simulink model "HANcoder_E407_KinematicAngleControl"  (R2022a)
settings: Solver=FixedStepDiscrete  StartTime=0.0  StopTime=1  FixedStep=0.01  RelTol=1e-3
PreLoadFcn:
  | librarySetup
  | eval([bdroot,'_startup']) %Calling [modelName]_startup.m
values from neighbouring files (symbols this model uses):
  L0b = 1    [HANcoder_E407_KinematicAngleControl_startup.m]    (also in HANcoder_E407_TTA_CombineModel_Membership_2022a_startup.m; HANcoder_E407_TTA_CombineModel_Membership_startup.m; HANcoder_E407_TTA_CombineModel_V2_startup.m; HANcoder_E407_TTA_CombineModel_startup.m)
  L0F = 3    [HANcoder_E407_KinematicAngleControl_startup.m]    (also in HANcoder_E407_TTA_CombineModel_Membership_2022a_startup.m; HANcoder_E407_TTA_CombineModel_Membership_startup.m; HANcoder_E407_TTA_CombineModel_V2_startup.m; HANcoder_E407_TTA_CombineModel_startup.m)
  L1F = 4    [HANcoder_E407_KinematicAngleControl_startup.m]    (also in HANcoder_E407_TTA_CombineModel_Membership_2022a_startup.m; HANcoder_E407_TTA_CombineModel_Membership_startup.m; HANcoder_E407_TTA_CombineModel_V2_startup.m; HANcoder_E407_TTA_CombineModel_startup.m)
  V2 = 1.3889    [HANcoder_E407_KinematicAngleControl_startup.m]    (also in HANcoder_E407_TTA_CombineModel_Membership_2022a_startup.m = 0.5; HANcoder_E407_TTA_CombineModel_Membership_startup.m = 0.5; HANcoder_E407_TTA_CombineModel_V2_startup.m = 0.5; HANcoder_E407_TTA_CombineModel_startup.m)
undefined symbols (not defined in the file or in its folder): A1, A2, A3, A4, A5, CON2, CON3, D4, D5
libraries: HANcoder_STM32_Target x14, slpidlib x1, simulink x1
settings Model: Creator=Jason van Kolfschoten  LastModifiedBy=lenovo
settings SolverCC: AlgebraicLoopSolver=TrustRegion  PositivePriorityOrder=on
settings DataIOCC: LimitDataPoints=on  SaveFormat=Array  SignalLoggingSaveFormat=ModelDataLogs  SaveOutput=off  SignalLogging=off  DSMLogging=off  SaveTime=off  ReturnWorkspaceOutputs=off
settings OptimizationCC: BlockReduction=off  DefaultParameterBehavior=Inlined  DefaultUnderspecifiedDataType=single  InlineInvariantSignals=on  ExpressionDepthLimit=2147483647  StateBitsets=on  DataBitsets=on  ZeroExternalMemoryAtStartup=off  ZeroInternalMemoryAtStartup=off  InitFltsAndDblsToZero=on  NoFixptDivByZeroProtection=on  EfficientFloat2IntCast=on  LifeSpan=inf  EfficientTunableParamExpr=on
settings DebuggingCC: SaveWithDisabledLinksMsg=none  SaveWithParameterizedLinksMsg=none  CheckSSInitialOutputMsg=off  UnderspecifiedInitializationDetection=Classic  MergeDetectMultiDrivingBlocksExec=none  SignalResolutionControl=TryResolveAll  SolverPrmCheckMsg=warning  InheritedTsInSrcMsg=none  MultiTaskDSMMsg=warning  MultiTaskCondExecSysMsg=none  ParameterPrecisionLossMsg=none  FcnCallInpInsideContextMsg=warning  UnconnectedInputMsg=warning  UnconnectedOutputMsg=warning  UnconnectedLineMsg=warning  StateNameClashWarn=warning  SFUnexpectedBacktrackingDiag=warning  SFNoUnconditionalDefaultTransitionDiag=warning  SFExecutionAtInitializationDiag=none  SFMachineParentedDataDiag=warning  ArithmeticOperatorsInVariantConditions=warning
settings HardwareCC: ProdBitPerPointer=32  ProdBitPerSizeT=32  ProdBitPerPtrDiffT=32  ProdLargestAtomicInteger=Long  ProdLargestAtomicFloat=Double  ProdWordSize=32  ProdHWDeviceType=ARM Compatible->ARM Cortex  TargetEndianess=LittleEndian  TargetHWDeviceType=Infineon->TriCore
settings ModelReferenceCC: PropagateSignalLabelsOutOfModel=off
settings SFSimCC: SimUseLocalCustomCode=off  MATLABDynamicMemAlloc=off  CustomCodeUndefinedFunction=UseInterfaceOnly
settings RTWCC: Description=Real-Time Workshop Embedded Coder (no auto configuration)  SystemTargetFile=ert.tlc  MakeCommand=make_rtw SHELL= HANcoder_PORTABLE=1 HANcoder_BOOTLOADER=1  TemplateMakefile=STM32_E407_gcc.tmf  RTWUseLocalCustomCode=off
settings CodeAppCC: ForceParamTrailComments=on  IgnoreCustomStorageClasses=off  SimulinkDataObjDesc=on  CustomSymbolStrGlobalVar=rt$N$M  CustomSymbolStrType=$N$M  CustomSymbolStrFcn=$N$M$F  CustomSymbolStrMacro=$N$M  InsertBlockDesc=on  StateflowObjectComments=on  InternalIdentifier=Classic
settings ERTTargetCC: TargetFcnLib=ansi_tfl_tmw.mat  MultiwordLength=2048  IncludeMdlTerminateFcn=off  SuppressErrorStatus=on  SupportNonFinite=off  GenerateASAP2=on  InlinedParameterPlacement=NonHierarchical  ERTCustomFileTemplate=example_file_process.tlc  ConvertIfToSwitch=off  SuppressUnreachableDefaultCases=off
settings ConfigComp: CovMetricSettings=dw  CovSaveCumulativeToWorkspaceVar=on  CovSaveSingleToWorkspaceVar=on  CovExternalEMLEnable=off  CovSFcnEnable=off  DVMaxProcessTime=600  DVAutomaticStubbing=off  DVModelCoverageObjectives=MCDC  DVMaxTestCaseSteps=500  DVTestSuiteOptimization=CombinedObjectives  DVDetectActiveLogic=on  DVSaveHarnessModel=on  DVHarnessSource=Signal Editor

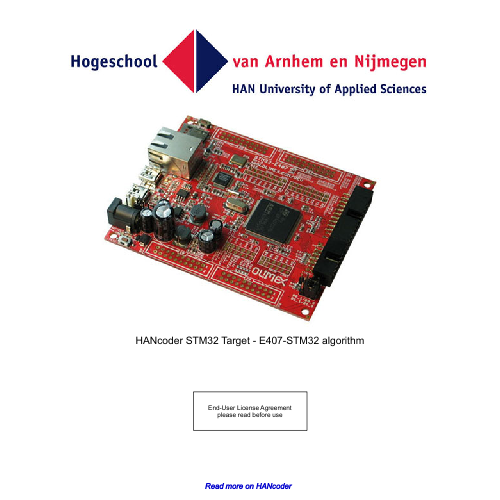
[thumbnail: Simulink's stored preview of the top-level diagram]
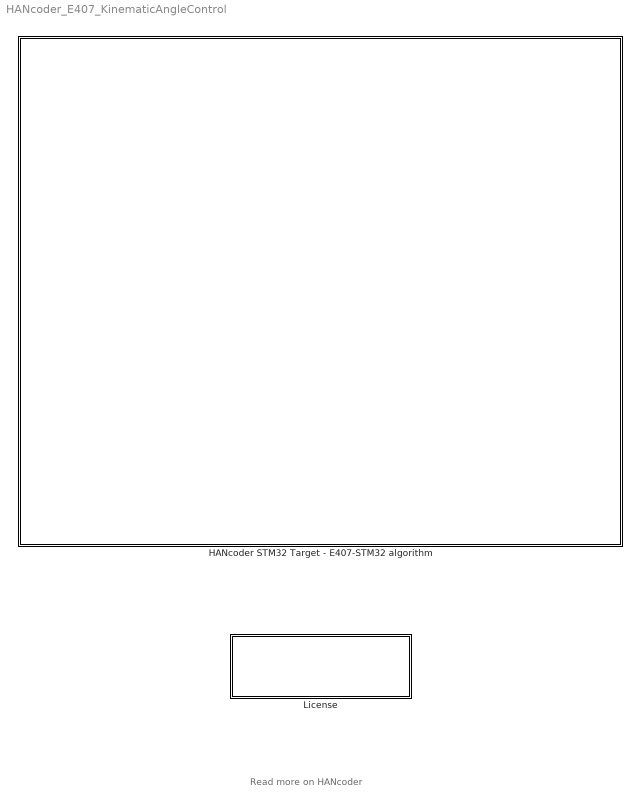
== system HANcoder_E407_KinematicAngleControl ==
  note: Read more on HANcoder
  HANcoder STM32 Target - E407-STM32 algorithm : Subsystem  mask(TopLevelSubsystem){}
      settings: CopyFcn=HANcoderChecks('Copy');  NameChangeFcn=HANcoderChecks('NameChangeE407');  MoveFcn=HANcoderChecks('MoveE407');
      mask Display: image(imread('STM32_E407_HAN.jpg'))
  License : Subsystem  mask(License){}
      settings: NameChangeFcn=HANcoderChecks('NameChangeLicenseBlock');  OpenFcn=winopen('License.pdf')  MoveFcn=HANcoderChecks('MoveLicenseBlock');
      mask Display: disp(['End-User License Agreement\n','please read before use']);

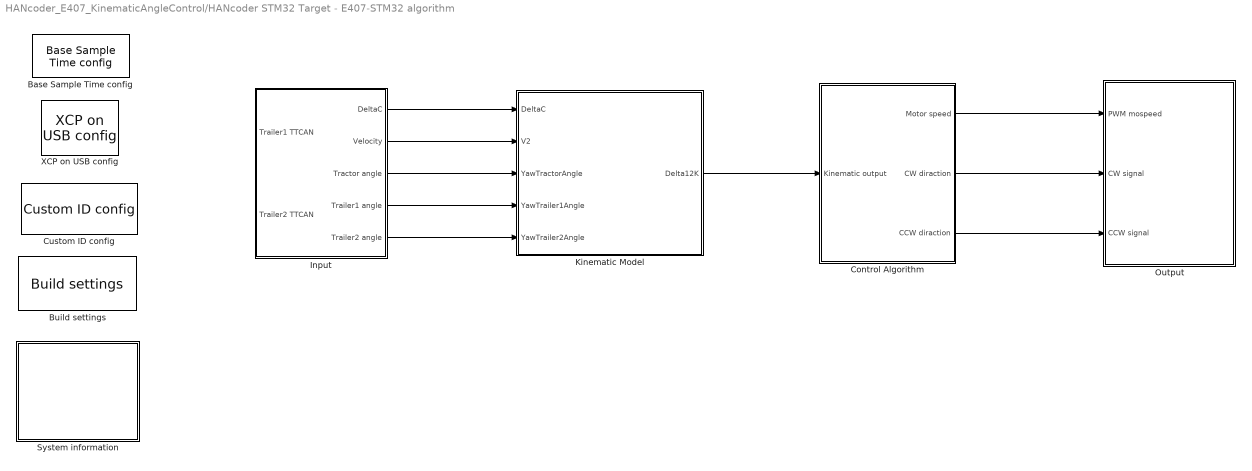
== system HANcoder_E407_KinematicAngleControl/HANcoder STM32 Target - E407-STM32 algorithm ==
  Base Sample Time config : HANcoder_STM32_Target/STM32-E407/System Config/Base Sample Time config  Tag=HANcoder_TARGET_STM32_E407  Description=HANcoder Target STM32-E407 blockset version 1.0  baseSampleTime=10  extraStack=100
      settings: SourceProductName=HANcoder STM32 Target
  Build settings : HANcoder_STM32_Target/STM32-E407/System Config/Build settings  Tag=HANcoder_TARGET_STM32_E407  AutoASAP2add=on  AutoFlash=USB
      settings: SourceProductName=HANcoder STM32 Target
  Control Algorithm : Subsystem
  Custom ID config : HANcoder_STM32_Target/STM32-E407/System Config/Custom ID config  Tag=HANcoder_TARGET_STM32_E407  softID=softwareID  softNUM=1
      settings: SourceProductName=HANcoder STM32 Target
  Input : Subsystem
  Kinematic Model : Subsystem
  "Output " : Subsystem
  System information : Subsystem
  XCP on USB config : HANcoder_STM32_Target/STM32-E407/System Config/XCP on USB config  Tag=HANcoder_TARGET_STM32_E407
      settings: SourceProductName=HANcoder STM32 Target
  wires:
  Input/1(DeltaC) -> Kinematic Model/1(DeltaC)
  Input/2(Velocity) -> Kinematic Model/2(V2)
  Input/3(Tractor angle) -> Kinematic Model/3(YawTractorAngle)
  Input/4(Trailer1 angle) -> Kinematic Model/4(YawTrailer1Angle)
  Input/5(Trailer2 angle) -> Kinematic Model/5(YawTrailer2Angle)
  Kinematic Model/1(Delta12K) -> Control Algorithm/1(Kinematic output)
  Control Algorithm/3(CCW diraction) -> "Output "/3(CCW signal)
  Control Algorithm/2(CW diraction) -> "Output "/2(CW signal)
  Control Algorithm/1(Motor speed) -> "Output "/1(PWM mospeed)

== system HANcoder_E407_KinematicAngleControl/License ==

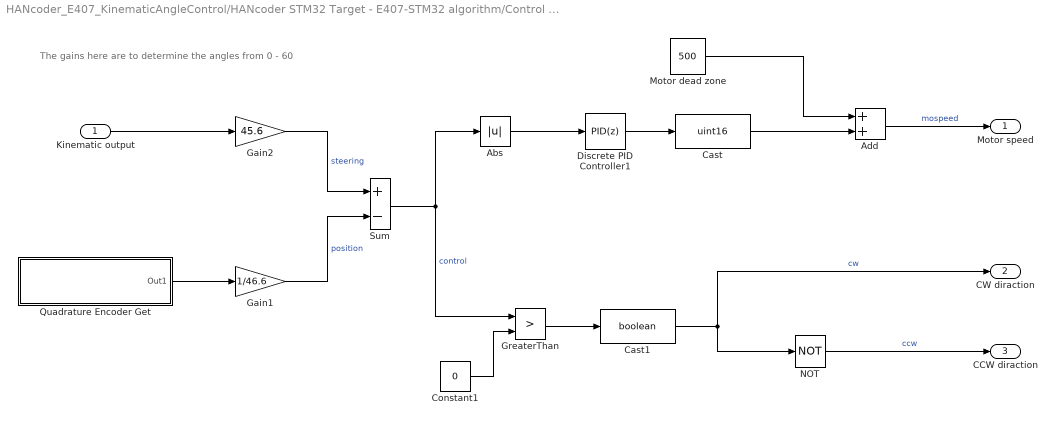
== system HANcoder_E407_KinematicAngleControl/HANcoder STM32 Target - E407-STM32 algorithm/Control Algorithm ==
  note: The gains here are to determine the angles from 0 - 60
  Kinematic output : Inport
  Abs : Abs  OutDataTypeStr=double  SaturateOnIntegerOverflow=off
  Add : Sum  AccumDataTypeStr=uint16
  Cast : DataTypeConversion  OutDataTypeStr=uint16  SaturateOnIntegerOverflow=off  RndMeth=Floor
  Cast1 : DataTypeConversion  OutDataTypeStr=boolean  SaturateOnIntegerOverflow=off  RndMeth=Floor
  Constant1 : Constant  Value=0
  Discrete PID Controller1 : slpidlib/PID Controller  Controller=PID  Form=Parallel  TimeDomain=Discrete-time  UseExternalTs=off  SampleTime=-1  IntegratorMethod=Forward Euler  FilterMethod=Forward Euler  ControllerParametersSource=internal  P=3  I=0.5  UseKiTs=off  D=0.5  N=100  UseFilter=on  TunerSelectOption=Transfer Function Based (PID Tuner App)  InitialConditionSource=internal  InitialConditionForIntegrator=0  InitialConditionForFilter=0  DifferentiatorICPrevScaledInput=0  ExternalReset=none  TrackingMode=off  Kt=1  LimitOutput=off  SatLimitsSource=internal  UpperSaturationLimit=inf  LowerSaturationLimit=-inf  LinearizeAsGain=off  AntiWindupMode=none  Kb=1  POutMin=[]  POutMax=[]  IOutMin=[]  IOutMax=[]  DOutMin=[]  DOutMax=[]  NOutMin=[]  NOutMax=[]  SumOutMin=[]  SumOutMax=[]  SaturationOutMin=[]  SaturationOutMax=[]  PParamMin=[]  PParamMax=[]  IParamMin=[]  IParamMax=[]  DParamMin=[]  DParamMax=[]  NParamMin=[]  NParamMax=[]  KbParamMin=[]  KbParamMax=[]  KtParamMin=[]  KtParamMax=[]  KbOutMin=[]  KbOutMax=[]  KtOutMin=[]  KtOutMax=[]  IntegratorOutMin=[]  IntegratorOutMax=[]  FilterOutMin=[]  FilterOutMax=[]  SumI1OutMin=[]  SumI1OutMax=[]  SumI2OutMin=[]  SumI2OutMax=[]  SumI3OutMin=[]  SumI3OutMax=[]  SumI4OutMin=[]  SumI4OutMax=[]  SumDOutMin=[]  SumDOutMax=[]  DifferentiatorOutMin=[]  DifferentiatorOutMax=[]  FilterDiffOutCoefMin=[]  FilterDiffOutCoefMax=[]  ReciprocalOutMin=[]  ReciprocalOutMax=[]  SumDenOutMin=[]  SumDenOutMax=[]  SumNumOutMin=[]  SumNumOutMax=[]  DivideOutMin=[]  DivideOutMax=[]  UdiffTsProdOutMin=[]  UdiffTsProdOutMax=[]  NTsProdOutMin=[]  NTsProdOutMax=[]  UintegralTsProdOutMin=[]  UintegralTsProdOutMax=[]  UngainTsProdOutMin=[]  UngainTsProdOutMax=[]  IntegratorContinuousStateAttributes=''  IntegratorStateMustResolveToSignalObject=off  IntegratorRTWStateStorageClass=Auto  FilterContinuousStateAttributes=''  FilterStateMustResolveToSignalObject=off  FilterRTWStateStorageClass=Auto  ParallelPVariant=InternalParameters  IdealPVariant=Disabled  IVariant=InternalParameters  DVariant=InternalParameters  IntegratorVariant=Discrete  SatVariant=Disabled  AWVariant=Passthrough  PCopyVariant=Disabled  TRVariant=Disabled  FdbkBlocksVariant=Forward  IdealPFdbkVariant=Disabled  SatFdbkVariant=Disabled  DerivativeFilterVariant=ForwardEulerFilter  NVariant=InternalParameters  NCopyVariant=Disabled  FilterICVariant=InternalICsFilter  IntegratorICVariant=InternalICs  ExternalResetVariant=Disabled  TRSumVariant=Passthrough  SumFdbkVariant=Disabled  SumVariant=Sum_PID  TsampFilterVariant=InternalTs  TsampNgainVariant=Passthrough  TsampIntegralVariant=Passthrough  ExternalSaturationOutDataTypeStr=Inherit: Same as second input  aMode=0
  Gain1 : Gain  Gain=1/46.6  OutDataTypeStr=double
  Gain2 : Gain  Gain=45.6
  GreaterThan : RelationalOperator  Operator=>  OutDataTypeStr=boolean  RndMeth=Simplest  InputSameDT=off
  Motor dead zone : Constant  Value=500  OutDataTypeStr=uint16
  NOT : Logic  Operator=NOT  IconShape=distinctive  AllPortsSameDT=off  OutDataTypeStr=boolean
  Quadrature Encoder Get : Subsystem  Tag=HANcoder_TARGET_STM32_E407  AncestorBlock=HANcoder_STM32_Target/STM32-E407/Timer Inputs/Quadrature Encoder Get  mask(Quadrature Encoder Inputs){moduleID=TIM3: CON4 - D12 & D11 (5V Tolerant), config=Floating, counterReset=off, tsamp=-1}
      mask prompts: moduleID "Quad encoder module"; config "Configuration"; counterReset "Show counter reset input"; tsamp "Sample time"
      mask help:
      | Function
      | ========
      | Reads the counter of the quadrature encoder module.
      |
      | Parameters
      | ==========
      | Quadrature encoder module:
      |   Selects the quadrature encoder module. The channel A and B signals of the
      |   encoder should be connected to the 2 input pins that belong to the module.
      |
      | Configuration:
      |   Determines if the input is floating or is connected to an internal
      |   pull-up or pull-down resistor.
      |
      | Show counter reset input:
      |   Configures if the input port for the counter reset should be shown.
      |
      |
      | Outport
      | ==========
      | 32-bit signed counter. The counter starts at zero and counts up or down
      | depending on the direction of the motor.
      mask init:
      | moduleIDInfoStr = sfcn_quad_encoder_get_mcb(2,moduleID, counterReset, config);
      settings: CopyFcn=sfcn_quad_encoder_get_chk();  MoveFcn=drawLogos
      mask Help: web('sfcn_quad_encoder_get.html');
      mask TypeOptions moduleID: TIM1: CON PE - 12 & 14 (5V Tolerant) | TIM3: CON4 - D12 & D11 (5V Tolerant) | TIM4: CON PD - 15 & 16 (5V Tolerant) | TIM8: UEXT - 3 & 4 (5V Tolerant)
      mask Callback moduleID: sfcn_quad_encoder_get_chk();
      mask TypeOptions config: Floating | Pullup | Pulldown
      mask Display: fprintf('Quad Encoder Get\n%s', moduleIDInfoStr);patch([135 141 141],[8 14 2],[1 0 0]);patch([143 143 149],[14 2 8],[0 0 0.35]);
  Sum : Sum  Inputs=+-
  Motor speed : Outport
  CW diraction : Outport  Port=2
  CCW diraction : Outport  Port=3
  wires:
  Motor dead zone/1 -> Add/1
  Sum/1 -> GreaterThan/1, Abs/1  "control"
  NOT/1 -> CCW diraction/1  "ccw"
  Abs/1 -> Discrete PID Controller1/1
  Cast/1 -> Add/2
  GreaterThan/1 -> Cast1/1
  Cast1/1 -> CW diraction/1, NOT/1  "cw"
  Add/1 -> Motor speed/1  "mospeed"
  Constant1/1 -> GreaterThan/2
  Gain1/1 -> Sum/2  "position"
  Discrete PID Controller1/1 -> Cast/1
  Quadrature Encoder Get/1(Out1) -> Gain1/1
  Gain2/1 -> Sum/1  "steering"
  Kinematic output/1 -> Gain2/1

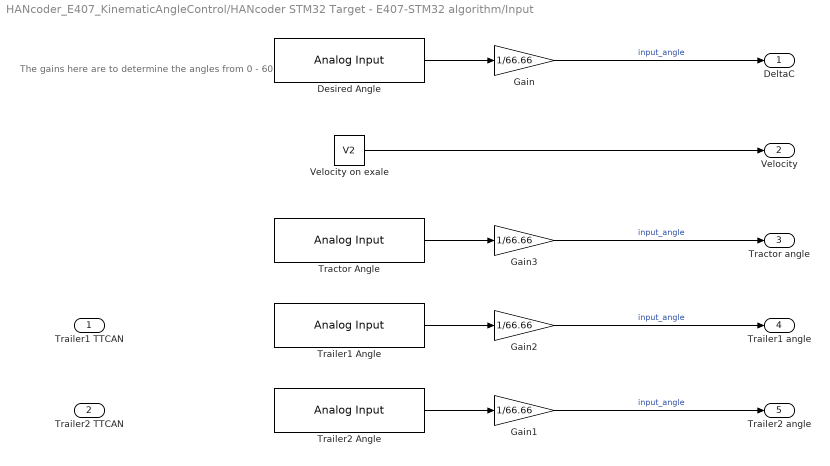
== system HANcoder_E407_KinematicAngleControl/HANcoder STM32 Target - E407-STM32 algorithm/Input ==
  note: The gains here are to determine the angles from 0 - 60
  Trailer1 TTCAN : Inport
  Trailer2 TTCAN : Inport  Port=2
  Desired Angle : HANcoder_STM32_Target/STM32-E407/Analog Inputs/Analog Input  Tag=HANcoder_TARGET_STM32_E407  pinID=CON2 - A1  tsamp=-1  filtered=off
      settings: SourceProductName=HANcoder STM32 Target
  Gain{,1..3} (4 alike) : Gain  Gain=1/66.66  OutDataTypeStr=double
  Tractor Angle : HANcoder_STM32_Target/STM32-E407/Analog Inputs/Analog Input  Tag=HANcoder_TARGET_STM32_E407  pinID=CON2 - A5  tsamp=-1  filtered=off
      settings: SourceProductName=HANcoder STM32 Target
  Trailer1 Angle : HANcoder_STM32_Target/STM32-E407/Analog Inputs/Analog Input  Tag=HANcoder_TARGET_STM32_E407  pinID=CON2 - A2  tsamp=-1  filtered=off
      settings: SourceProductName=HANcoder STM32 Target
  Trailer2 Angle : HANcoder_STM32_Target/STM32-E407/Analog Inputs/Analog Input  Tag=HANcoder_TARGET_STM32_E407  pinID=CON2 - A3  tsamp=-1  filtered=off
      settings: SourceProductName=HANcoder STM32 Target
  Velocity on exale : Constant  Value=V2
  DeltaC : Outport
  Velocity : Outport  Port=2
  Tractor angle : Outport  Port=3
  Trailer1 angle : Outport  Port=4
  Trailer2 angle : Outport  Port=5
  wires:
  Velocity on exale/1 -> Velocity/1
  Desired Angle/1 -> Gain/1
  Gain/1 -> DeltaC/1  "input_angle"
  Gain3/1 -> Tractor angle/1  "input_angle"
  Tractor Angle/1 -> Gain3/1
  Gain2/1 -> Trailer1 angle/1  "input_angle"
  Trailer1 Angle/1 -> Gain2/1
  Gain1/1 -> Trailer2 angle/1  "input_angle"
  Trailer2 Angle/1 -> Gain1/1

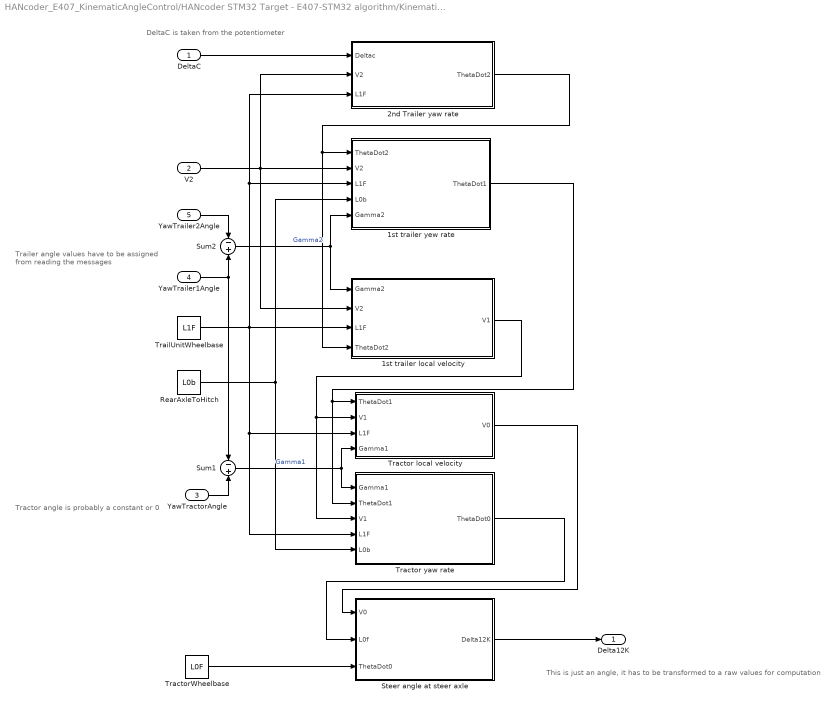
== system HANcoder_E407_KinematicAngleControl/HANcoder STM32 Target - E407-STM32 algorithm/Kinematic Model ==
  note: This is just an angle, it has to be transformed to a raw values for computation
  note: Trailer angle values have to be assigned
      |  from reading the messages
  note: Tractor angle is probably a constant or 0
  note: DeltaC is taken from the potentiometer
  DeltaC : Inport
  V2 : Inport  Port=2
  YawTractorAngle : Inport  Port=3
  YawTrailer1Angle : Inport  Port=4
  YawTrailer2Angle : Inport  Port=5
  1st trailer local velocity : Subsystem
  1st trailer yew rate : Subsystem
  2nd Trailer yaw rate : Subsystem
  RearAxleToHitch : Constant  Value=L0b
  Steer angle at steer axle : Subsystem
  Sum1 : Sum  Inputs=-+
  Sum2 : Sum  Inputs=-+
  Tractor local velocity : Subsystem
  Tractor yaw rate : Subsystem
  TractorWheelbase : Constant  Value=L0F
  TrailUnitWheelbase : Constant  Value=L1F
  Delta12K : Outport
  wires:
  TractorWheelbase/1 -> Steer angle at steer axle/3(ThetaDot0)
  YawTractorAngle/1 -> Sum1/2
  Sum2/1 -> 1st trailer local velocity/1(Gamma2), 1st trailer yew rate/5(Gamma2)  "Gamma2"
  Steer angle at steer axle/1(Delta12K) -> Delta12K/1
  Sum1/1 -> Tractor yaw rate/1(Gamma1), Tractor local velocity/4(Gamma1)  "Gamma1"
  DeltaC/1 -> 2nd Trailer yaw rate/1(Deltac)
  YawTrailer2Angle/1 -> Sum2/1
  TrailUnitWheelbase/1 -> Tractor yaw rate/4(L1F), Tractor local velocity/3(L1F), 1st trailer local velocity/3(L1F), 1st trailer yew rate/3(L1F), 2nd Trailer yaw rate/3(L1F)
  V2/1 -> 1st trailer yew rate/2(V2), 1st trailer local velocity/2(V2), 2nd Trailer yaw rate/2(V2)
  1st trailer local velocity/1(V1) -> Tractor yaw rate/3(V1), Tractor local velocity/2(V1)
  RearAxleToHitch/1 -> Tractor yaw rate/5(L0b), 1st trailer yew rate/4(L0b)
  YawTrailer1Angle/1 -> Sum1/1, Sum2/2
  Tractor local velocity/1(V0) -> Steer angle at steer axle/1(V0)
  Tractor yaw rate/1(ThetaDot0) -> Steer angle at steer axle/2(L0f)
  1st trailer yew rate/1(ThetaDot1) -> Tractor yaw rate/2(ThetaDot1), Tractor local velocity/1(ThetaDot1)
  2nd Trailer yaw rate/1(ThetaDot2) -> 1st trailer local velocity/4(ThetaDot2), 1st trailer yew rate/1(ThetaDot2)

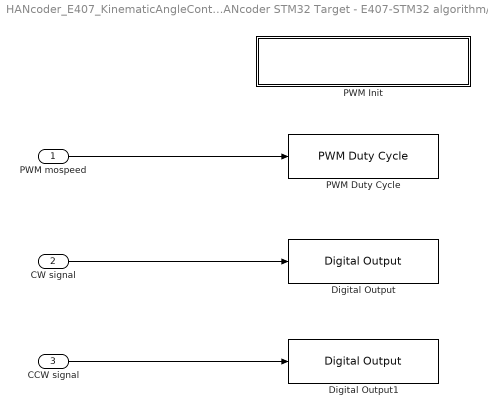
== system HANcoder_E407_KinematicAngleControl/HANcoder STM32 Target - E407-STM32 algorithm/Output  ==
  PWM mospeed : Inport
  CW signal : Inport  Port=2
  CCW signal : Inport  Port=3
  Digital Output : HANcoder_STM32_Target/STM32-E407/Digital Outputs/Digital Output  Tag=HANcoder_TARGET_STM32_E407  pinID=CON3 - D4  config=Push pull  tsamp=-1
      settings: SourceProductName=HANcoder STM32 Target
  Digital Output1 : HANcoder_STM32_Target/STM32-E407/Digital Outputs/Digital Output  Tag=HANcoder_TARGET_STM32_E407  pinID=CON3 - D5  config=Push pull  tsamp=-1
      settings: SourceProductName=HANcoder STM32 Target
  PWM Duty Cycle : HANcoder_STM32_Target/STM32-E407/PWM Outputs/PWM Duty Cycle  Tag=HANcoder_TARGET_STM32_E407  pinID=CON2 - A4  tsamp=-1
      settings: SourceProductName=HANcoder STM32 Target
  PWM Init : Subsystem  Tag=HANcoder_TARGET_STM32_E407  AncestorBlock=HANcoder_STM32_Target/STM32-E407/PWM Outputs/PWM Init  mask(Pulse Width Modulation Initialization){moduleID=TIM14: A4 & n/a & n/a & n/a, frequency=10253, alignment=Edge aligned, enableIRQoutput=off, ch1On=on, ch1Pol=Active high, ch1Inv=off, ch2On=on, ch2Pol=Active high, ch2Inv=off, ch3On=off, ch3Pol=Active high, ch3Inv=off, ch4On=off, ch4Pol=Active high, ch4Inv=off}
      mask prompts: moduleID "PWM module"; frequency "Signal frequency [Hz]"; alignment "Signal alignment"; enableIRQoutput "Enable IRQ output"; ch1On "Generate PWM signal on channel 1"; ch1Pol "Select signal polarity"; ch1Inv "Enable inverted signal on additional output pin"; ch2On "Generate PWM signal on channel 2"; ch2Pol "Select signal polarity"; ch2Inv "Enable inverted signal on additional output pin"; ch3On "Generate PWM signal on channel 3"; ch3Pol "Select signal polarity"; ch3Inv "Enable inverted signal on additional output pin"; ch4On "Generate PWM signal on channel 4"; ch4Pol "Select signal polarity"; ch4Inv "Enable inverted signal on additional output pin"
      mask help:
      | Function
      | ========
      | A 'PWM Init' block configures one of the STM32 timer modules for PWM
      | functionality, allowing a PWM signal to be generated on up to 4 timer
      | channels and their associated output pins.
      |
      | Parameters
      | ==========
      | General - PWM module:
      |   Select the PWM module to use. The name in the combo box contains
      |   information about which pins on the target belong to this timer module.
      |   Also the first pin corresponds with the first channel and so on:
      |   TIMx: Ch1 & Ch2 & Ch3...
      |
      | General - Signal frequency:
      |   Determines the signal frequency in Hz. If you click 'Apply' after entering
      |   the desired frequency it will automatically be adjusted to the closest
      |   supported value.
      |
      | General - Signal Aligment:
      |   Determines the aligment of the signal. It can either be edge aligned or
      |   center aligned.
      |
      | General - Enable IRQ output
      |   Controls whether or not the IRQ output is available.
      |
      | Channel x - Generate PWM signal on channel x:
      |   Enable to configure the channel for PWM functionality so that the PWM signal
      |   is outputted on the channel's associated microcontroller pin.
      |
      | Channel x - Signal polarity:
      |   Selects the polarity of the signal.
      |
      | Channel x - Enable inverted signal on additional output pin:
      |   When enabled, a second PWM signal will be generated on an additional
      |   microcontroller pin where the signal is an exact inversion of the first signal.
      mask init:
      | moduleIDInfoStr = sfcn_pwmout_init_mcb(2, moduleID, frequency, alignment, enableIRQoutput, ch1On, ch2On, ch3On, ch4On, ch1Pol, ch2Pol, ch3Pol, ch4Pol, ch1Inv, ch2Inv, ch3Inv, ch4Inv);
      settings: CopyFcn=sfcn_pwmout_init_chk();  MoveFcn=drawLogos
      mask Help: web('sfcn_pwmout_init.html');
      mask TypeOptions moduleID: TIM1:   PE12 & PE14 & PE16 & PE17 + N-channels PE11 & PE13 & PE15 | TIM2:   D13 & n/a & n/a & n/a | TIM3:   D12 & D11 & n/a & n/a | TIM4:   PD15 & PD16 &n/a & n/a | TIM8:   UEXT3 & UEXT4 & n/a & n/a | TIM9:   D4 & D5 & n/a & n/a | TIM10: A1 & n/a & n/a & n/a | TIM11: A2 & n/a & n/a & n/a | TIM13: A3 & n/a & n/a & n/a | TIM14: A4 & n/a & n/a & n/a
      mask Callback moduleID: sfcn_pwmout_init_chk();
      mask TypeOptions alignment: Edge aligned | Center aligned
      mask TypeOptions ch1Pol: Active high | Active low
      mask TypeOptions ch2Pol: Active high | Active low
      mask TypeOptions ch3Pol: Active high | Active low
      mask TypeOptions ch4Pol: Active high | Active low
      mask Display: fprintf('PWM Init\n%s', moduleIDInfoStr);patch([195 201 201],[8 14 2],[1 0 0]);patch([203 203 209],[14 2 8],[0 0 0.35]);
  wires:
  PWM mospeed/1 -> PWM Duty Cycle/1
  CW signal/1 -> Digital Output/1
  CCW signal/1 -> Digital Output1/1

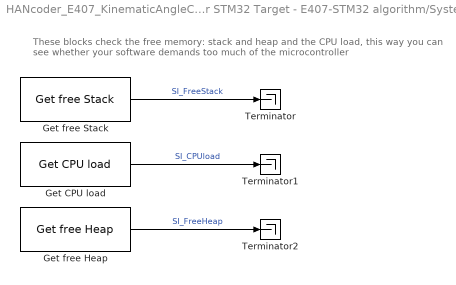
== system HANcoder_E407_KinematicAngleControl/HANcoder STM32 Target - E407-STM32 algorithm/System information ==
  note: These blocks check the free memory: stack and heap and the CPU load,
      | this way you can see whether your software demands too much of the microcontroller
  Get CPU load : HANcoder_STM32_Target/STM32-E407/System Management/Get CPU load  Tag=HANcoder_TARGET_STM32_E407  mode=Current CPU load  tsamp=-1
      settings: SourceProductName=HANcoder STM32 Target
  Get free Heap : HANcoder_STM32_Target/STM32-E407/System Management/Get free Heap  Tag=HANcoder_TARGET_STM32_E407  tsamp=-1
      settings: SourceProductName=HANcoder STM32 Target
  Get free Stack : HANcoder_STM32_Target/STM32-E407/System Management/Get free Stack  Tag=HANcoder_TARGET_STM32_E407  taskIdx=Application Control Task  tsamp=-1
      settings: SourceProductName=HANcoder STM32 Target
  Terminator : Terminator
  Terminator1 : Terminator
  Terminator2 : Terminator
  wires:
  Get CPU load/1 -> Terminator1/1  "SI_CPUload"
  Get free Stack/1 -> Terminator/1  "SI_FreeStack"
  Get free Heap/1 -> Terminator2/1  "SI_FreeHeap"

== system HANcoder_E407_KinematicAngleControl/HANcoder STM32 Target - E407-STM32 algorithm/Control Algorithm/Quadrature Encoder Get ==
  Data Type Conversion : DataTypeConversion  OutDataTypeStr=boolean  SaturateOnIntegerOverflow=off  RndMeth=Floor
  Detect Increase : simulink/Logic and Bit Operations/Detect Increase  vinit=0.0  OutDataTypeStr=uint8
  Gnd1 : Ground
  Level-2 M-file S-Function : M-S-Function  FunctionName=sfcn_quad_encoder_get  Parameters=tsamp, moduleID
  Out1 : Outport
  wires:
  Level-2 M-file S-Function/1 -> Out1/1
  Gnd1/1 -> Detect Increase/1
  Detect Increase/1 -> Data Type Conversion/1
  Data Type Conversion/1 -> Level-2 M-file S-Function/1

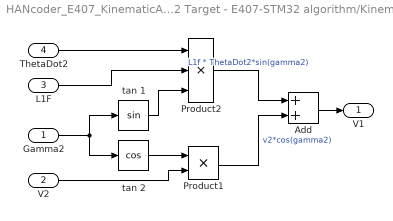
== system HANcoder_E407_KinematicAngleControl/HANcoder STM32 Target - E407-STM32 algorithm/Kinematic Model/1st trailer local velocity ==
  Gamma2 : Inport
  V2 : Inport  Port=2
  L1F : Inport  Port=3
  ThetaDot2 : Inport  Port=4
  Add : Sum
  Product1 : Product  Inputs=**
  Product2 : Product  Inputs=***
  tan 1 : Trigonometry
  tan 2 : Trigonometry  Operator=cos
  V1 : Outport
  wires:
  tan 1/1 -> Product2/3
  tan 2/1 -> Product1/1
  Gamma2/1 -> tan 1/1, tan 2/1
  L1F/1 -> Product2/2
  V2/1 -> Product1/2
  Product2/1 -> Add/1  "L1f * ThetaDot2*sin(gamma2)"
  Product1/1 -> Add/2  "v2*cos(gamma2)"
  Add/1 -> V1/1
  ThetaDot2/1 -> Product2/1

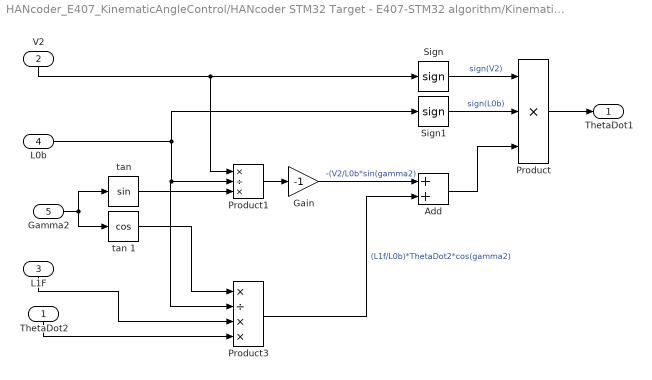
== system HANcoder_E407_KinematicAngleControl/HANcoder STM32 Target - E407-STM32 algorithm/Kinematic Model/1st trailer yew rate ==
  ThetaDot2 : Inport
  V2 : Inport  Port=2
  L1F : Inport  Port=3
  L0b : Inport  Port=4
  Gamma2 : Inport  Port=5
  Add : Sum
  Gain : Gain  Gain=-1
  Product : Product  Inputs=***
  Product1 : Product  Inputs=*/*
  Product3 : Product  Inputs=*/**
  Sign : Signum
  Sign1 : Signum
  "tan " : Trigonometry
  tan 1 : Trigonometry  Operator=cos
  ThetaDot1 : Outport
  wires:
  V2/1 -> Product1/1, Sign/1
  L1F/1 -> Product3/3
  ThetaDot2/1 -> Product3/4
  Product3/1 -> Add/2  "(L1f/L0b)*ThetaDot2*cos(gamma2)"
  Product1/1 -> Gain/1
  Sign/1 -> Product/1  "sign(V2)"
  Gamma2/1 -> "tan "/1, tan 1/1
  Add/1 -> Product/3
  Sign1/1 -> Product/2  "sign(L0b)"
  Gain/1 -> Add/1  "-(V2/L0b*sin(gamma2)"
  Product/1 -> ThetaDot1/1
  L0b/1 -> Product1/2, Product3/2, Sign1/1
  tan 1/1 -> Product3/1
  "tan "/1 -> Product1/3

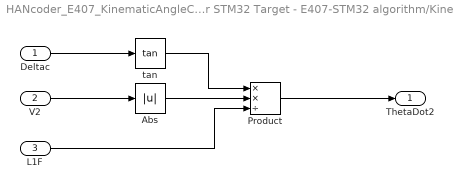
== system HANcoder_E407_KinematicAngleControl/HANcoder STM32 Target - E407-STM32 algorithm/Kinematic Model/2nd Trailer yaw rate ==
  Deltac : Inport
  V2 : Inport  Port=2
  L1F : Inport  Port=3
  Abs : Abs  SaturateOnIntegerOverflow=off
  Product : Product  Inputs=**/
  "tan " : Trigonometry  Operator=tan
  ThetaDot2 : Outport
  wires:
  "tan "/1 -> Product/1
  Product/1 -> ThetaDot2/1
  Abs/1 -> Product/2
  V2/1 -> Abs/1
  L1F/1 -> Product/3
  Deltac/1 -> "tan "/1

== system HANcoder_E407_KinematicAngleControl/HANcoder STM32 Target - E407-STM32 algorithm/Kinematic Model/Steer angle at steer axle ==
  V0 : Inport
  L0f : Inport  Port=2
  ThetaDot0 : Inport  Port=3
  Product1 : Product  Inputs=**/
  tan 1 : Trigonometry  Operator=atan
  Delta12K : Outport
  wires:
  Product1/1 -> tan 1/1
  tan 1/1 -> Delta12K/1
  L0f/1 -> Product1/1
  V0/1 -> Product1/3
  ThetaDot0/1 -> Product1/2

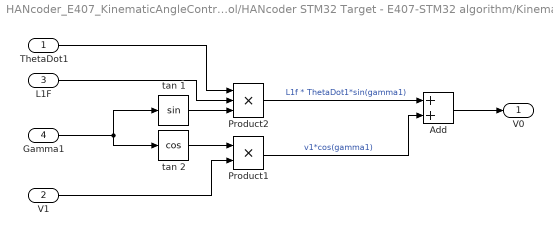
== system HANcoder_E407_KinematicAngleControl/HANcoder STM32 Target - E407-STM32 algorithm/Kinematic Model/Tractor local velocity ==
  ThetaDot1 : Inport
  V1 : Inport  Port=2
  L1F : Inport  Port=3
  Gamma1 : Inport  Port=4
  Add : Sum
  Product1 : Product  Inputs=**
  Product2 : Product  Inputs=***
  tan 1 : Trigonometry
  tan 2 : Trigonometry  Operator=cos
  V0 : Outport
  wires:
  Gamma1/1 -> tan 1/1, tan 2/1
  Product1/1 -> Add/2  "v1*cos(gamma1)"
  Product2/1 -> Add/1  "L1f * ThetaDot1*sin(gamma1)"
  Add/1 -> V0/1
  tan 2/1 -> Product1/1
  tan 1/1 -> Product2/3
  V1/1 -> Product1/2
  ThetaDot1/1 -> Product2/1
  L1F/1 -> Product2/2

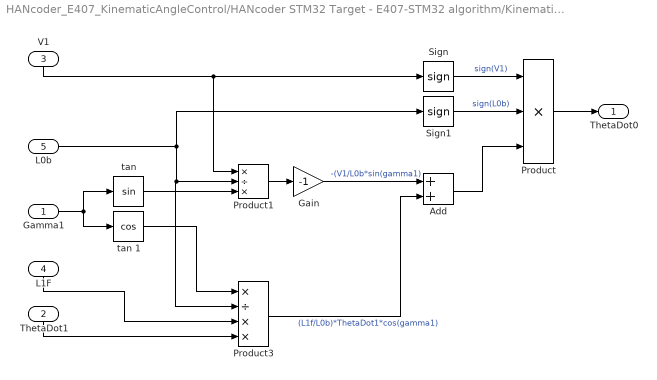
== system HANcoder_E407_KinematicAngleControl/HANcoder STM32 Target - E407-STM32 algorithm/Kinematic Model/Tractor yaw rate ==
  Gamma1 : Inport
  ThetaDot1 : Inport  Port=2
  V1 : Inport  Port=3
  L1F : Inport  Port=4
  L0b : Inport  Port=5
  Add : Sum
  Gain : Gain  Gain=-1
  Product : Product  Inputs=***
  Product1 : Product  Inputs=*/*
  Product3 : Product  Inputs=*/**
  Sign : Signum
  Sign1 : Signum
  "tan " : Trigonometry
  tan 1 : Trigonometry  Operator=cos
  ThetaDot0 : Outport
  wires:
  V1/1 -> Product1/1, Sign/1
  L1F/1 -> Product3/3
  ThetaDot1/1 -> Product3/4
  Product3/1 -> Add/2  "(L1f/L0b)*ThetaDot1*cos(gamma1)"
  Product1/1 -> Gain/1
  Sign/1 -> Product/1  "sign(V1)"
  Gamma1/1 -> "tan "/1, tan 1/1
  Add/1 -> Product/3
  Sign1/1 -> Product/2  "sign(L0b)"
  Gain/1 -> Add/1  "-(V1/L0b*sin(gamma1)"
  Product/1 -> ThetaDot0/1
  L0b/1 -> Sign1/1, Product1/2, Product3/2
  tan 1/1 -> Product3/1
  "tan "/1 -> Product1/3

== system HANcoder_E407_KinematicAngleControl/HANcoder STM32 Target - E407-STM32 algorithm/Output /PWM Init ==
  S-Function : S-Function  FunctionName=sfcn_pwmout_init  SFunctionDeploymentMode=off  EnableBusSupport=off
  Term1 : Terminator
  wires:
  S-Function/1 -> Term1/1
